simulink model "bdot_simple_sim"  (R2016b)
settings: Solver=VariableStepAuto  StartTime=0.0  StopTime=10000  RelTol=1e-3  EnableMultiTasking=on
values from neighbouring files (symbols this model uses):
  fsw_params = init_fsw_params()    [bdot_controller_edit_test.m]    (also in bdot_controlller_unit_test.m)
  sim_params = init_sim_params(fsw_params)    [bdot_controller_edit_test.m]    (also in bdot_controlller_unit_test.m)
undefined symbols (not defined in the file or in its folder): DiscIntNeverNeededParam
libraries: aerolibutil x5, vrlib x1, bdot_controller_lib x1, magnetorquer_assembly_lib x1
settings Model: Creator=Taylor  LastModifiedBy=taylorreynolds
settings OptimizationCC: LifeSpan=inf
settings DebuggingCC: SFUnexpectedBacktrackingDiag=warning  SFNoUnconditionalDefaultTransitionDiag=warning  SFExecutionAtInitializationDiag=none
settings GRTTargetCC: TargetLangStandard=C89/C90 (ANSI)  GeneratePreprocessorConditionals=Disable all
settings ConfigComp: CovMetricSettings=dw  CovHtmlReporting=on  CovSaveCumulativeToWorkspaceVar=on  CovSaveSingleToWorkspaceVar=on  CovExternalEMLEnable=off

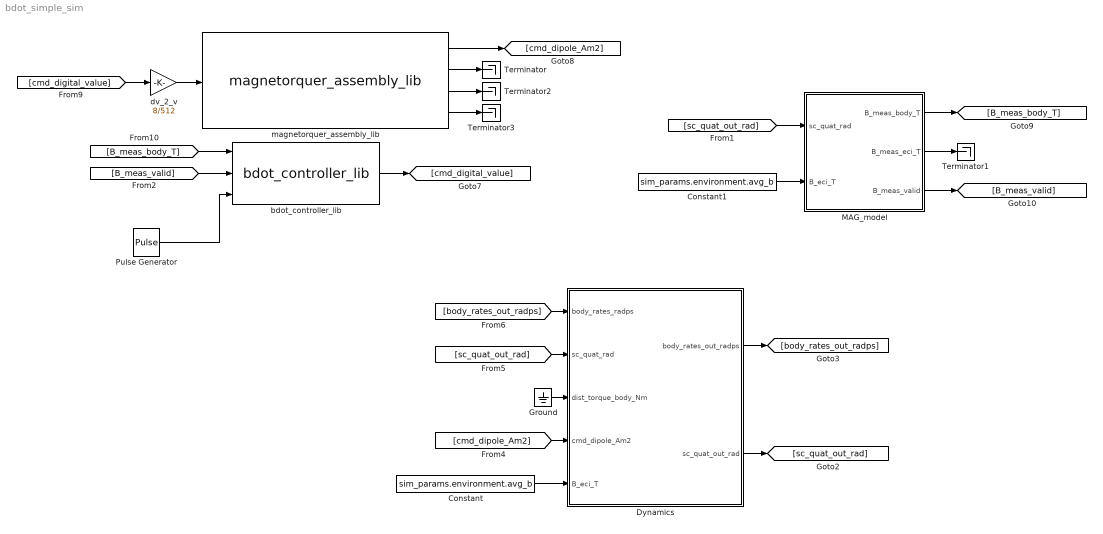
== system bdot_simple_sim ==
  Constant : Constant  Value=sim_params.environment.avg_b
  Constant1 : Constant  Value=sim_params.environment.avg_b
  Dynamics : Subsystem
  Ground : Ground
  MAG_model : Subsystem
  Pulse Generator : DiscretePulseGenerator  PulseType=Time based  Period=1  PulseWidth=sim_params.actuators.magnetorquer.actuation_time_pct
  Terminator{,1..3} (4 alike) : Terminator
  bdot_controller_lib : bdot_controller_lib/bdot_controller_lib
  dv_2_v : Gain  Gain=8/512
  magnetorquer_assembly_lib : magnetorquer_assembly_lib/magnetorquer_assembly_lib
  wires:
  bdot_controller_lib/1 -> [cmd_digital_value]
  [B_meas_body_T] -> bdot_controller_lib/1
  MAG_model/3(B_meas_valid) -> [B_meas_valid]
  MAG_model/1(B_meas_body_T) -> [B_meas_body_T]
  MAG_model/2(B_meas_eci_T) -> Terminator1/1
  [sc_quat_out_rad] -> MAG_model/1(sc_quat_rad)
  Constant1/1 -> MAG_model/2(B_eci_T)
  [body_rates_out_radps] -> Dynamics/1(body_rates_radps)
  Dynamics/1(body_rates_out_radps) -> [body_rates_out_radps]
  Dynamics/2(sc_quat_out_rad) -> [sc_quat_out_rad]
  [sc_quat_out_rad] -> Dynamics/2(sc_quat_rad)
  Ground/1 -> Dynamics/3(dist_torque_body_Nm)
  [cmd_dipole_Am2] -> Dynamics/4(cmd_dipole_Am2)
  Constant/1 -> Dynamics/5(B_eci_T)
  [B_meas_valid] -> bdot_controller_lib/2
  Pulse Generator/1 -> bdot_controller_lib/3
  dv_2_v/1 -> magnetorquer_assembly_lib/1
  [cmd_digital_value] -> dv_2_v/1
  magnetorquer_assembly_lib/1 -> [cmd_dipole_Am2]
  magnetorquer_assembly_lib/2 -> Terminator/1
  magnetorquer_assembly_lib/4 -> Terminator3/1
  magnetorquer_assembly_lib/3 -> Terminator2/1

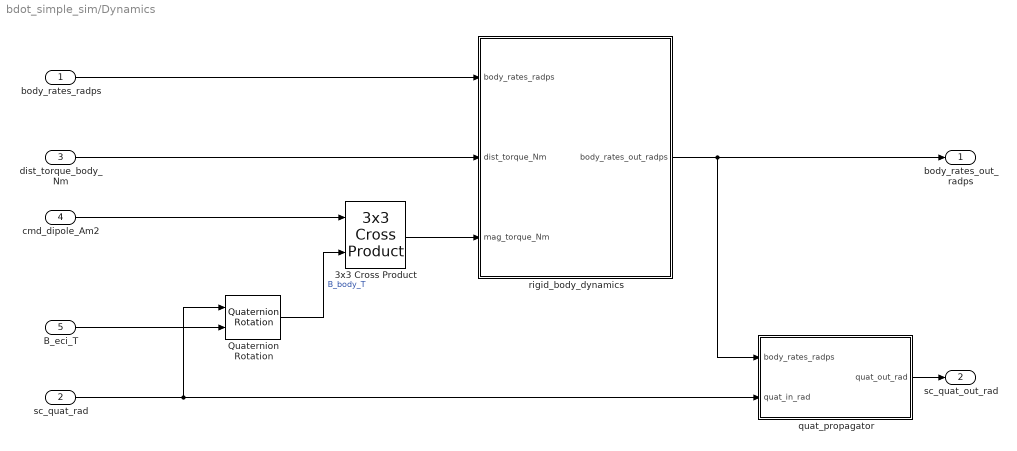
== system bdot_simple_sim/Dynamics ==
  body_rates_radps : Inport
  sc_quat_rad : Inport  Port=2
  dist_torque_body_Nm : Inport  Port=3
  cmd_dipole_Am2 : Inport  Port=4
  B_eci_T : Inport  Port=5
  3x3 Cross Product : aerolibutil/3x3 Cross Product
  Quaternion Rotation : aerolibutil/Quaternion Rotation
  quat_propagator : Subsystem
  rigid_body_dynamics : Subsystem
  body_rates_out_radps : Outport
  sc_quat_out_rad : Outport  Port=2
  wires:
  Quaternion Rotation/1 -> 3x3 Cross Product/2  "B_body_T"
  cmd_dipole_Am2/1 -> 3x3 Cross Product/1
  dist_torque_body_Nm/1 -> rigid_body_dynamics/2(dist_torque_Nm)
  sc_quat_rad/1 -> Quaternion Rotation/1, quat_propagator/2(quat_in_rad)
  quat_propagator/1(quat_out_rad) -> sc_quat_out_rad/1
  body_rates_radps/1 -> rigid_body_dynamics/1(body_rates_radps)
  rigid_body_dynamics/1(body_rates_out_radps) -> body_rates_out_radps/1, quat_propagator/1(body_rates_radps)
  B_eci_T/1 -> Quaternion Rotation/2
  3x3 Cross Product/1 -> rigid_body_dynamics/3(mag_torque_Nm)

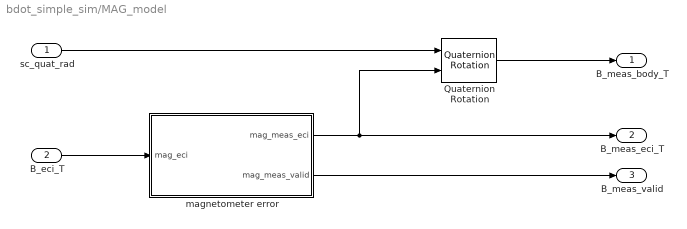
== system bdot_simple_sim/MAG_model ==
  sc_quat_rad : Inport
  B_eci_T : Inport  Port=2
  Quaternion Rotation : aerolibutil/Quaternion Rotation
  magnetometer error : Subsystem
  B_meas_body_T : Outport
  B_meas_eci_T : Outport  Port=2
  B_meas_valid : Outport  Port=3
  wires:
  sc_quat_rad/1 -> Quaternion Rotation/1
  B_eci_T/1 -> magnetometer error/1(mag_eci)
  magnetometer error/1(mag_meas_eci) -> Quaternion Rotation/2, B_meas_eci_T/1
  Quaternion Rotation/1 -> B_meas_body_T/1
  magnetometer error/2(mag_meas_valid) -> B_meas_valid/1

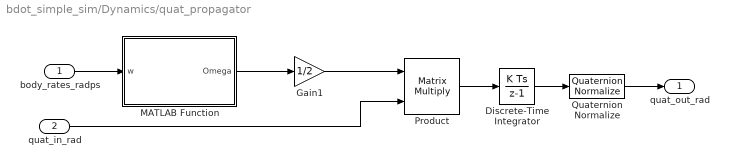
== system bdot_simple_sim/Dynamics/quat_propagator ==
  body_rates_radps : Inport
  quat_in_rad : Inport  Port=2
  Discrete-Time Integrator : DiscreteIntegrator  InitialCondition=sim_params.dynamics.ic.quat_init  InitialConditionSetting=State (most efficient)  SampleTime=fsw_params.sample_time_s  ICPrevOutput=DiscIntNeverNeededParam  ICPrevScaledInput=DiscIntNeverNeededParam
  Gain1 : Gain  Gain=1/2
  MATLAB Function : MATLAB Function  TreatAsAtomicUnit=on
  Product : Product  Multiplication=Matrix(*)  RndMeth=Zero
  Quaternion Normalize : aerolibutil/Quaternion Normalize
  quat_out_rad : Outport
  wires:
  Product/1 -> Discrete-Time Integrator/1
  Quaternion Normalize/1 -> quat_out_rad/1
  Discrete-Time Integrator/1 -> Quaternion Normalize/1
  Gain1/1 -> Product/1
  quat_in_rad/1 -> Product/2
  body_rates_radps/1 -> MATLAB Function/1(w)
  MATLAB Function/1(Omega) -> Gain1/1

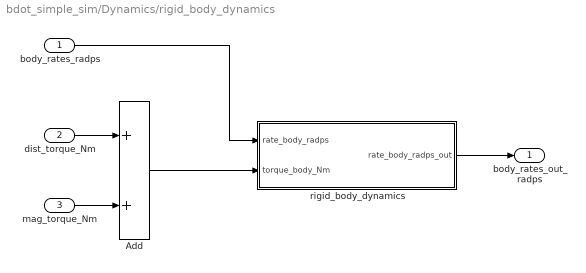
== system bdot_simple_sim/Dynamics/rigid_body_dynamics ==
  body_rates_radps : Inport
  dist_torque_Nm : Inport  Port=2
  mag_torque_Nm : Inport  Port=3
  Add : Sum
  rigid_body_dynamics : Subsystem
  body_rates_out_radps : Outport
  wires:
  dist_torque_Nm/1 -> Add/1
  Add/1 -> rigid_body_dynamics/2(torque_body_Nm)
  mag_torque_Nm/1 -> Add/2
  rigid_body_dynamics/1(rate_body_radps_out) -> body_rates_out_radps/1
  body_rates_radps/1 -> rigid_body_dynamics/1(rate_body_radps)

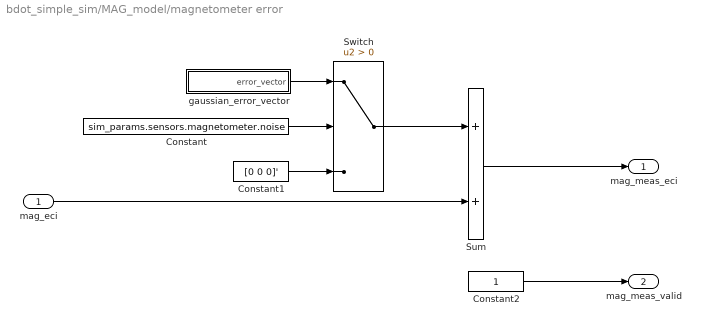
== system bdot_simple_sim/MAG_model/magnetometer error ==
  mag_eci : Inport
  Constant : Constant  Value=sim_params.sensors.magnetometer.noise
  Constant1 : Constant  Value=[0 0 0]'
  Constant2 : Constant
  Sum : Sum
  Switch : Switch  Criteria=u2 > Threshold
  gaussian_error_vector : Subsystem
  mag_meas_eci : Outport
  mag_meas_valid : Outport  Port=2
  wires:
  Constant2/1 -> mag_meas_valid/1
  Switch/1 -> Sum/1
  Constant1/1 -> Switch/3
  Constant/1 -> Switch/2
  gaussian_error_vector/1(error_vector) -> Switch/1
  Sum/1 -> mag_meas_eci/1
  mag_eci/1 -> Sum/2

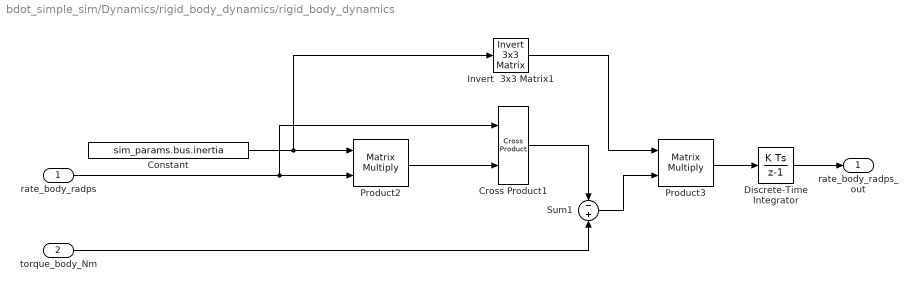
== system bdot_simple_sim/Dynamics/rigid_body_dynamics/rigid_body_dynamics ==
  rate_body_radps : Inport
  torque_body_Nm : Inport  Port=2
  Constant : Constant  Value=sim_params.bus.inertia
  Cross Product1 : vrlib/Utilities/Cross Product
  Discrete-Time Integrator : DiscreteIntegrator  InitialCondition=sim_params.dynamics.ic.rate_init  InitialConditionSetting=State (most efficient)  SampleTime=fsw_params.sample_time_s  ICPrevOutput=DiscIntNeverNeededParam  ICPrevScaledInput=DiscIntNeverNeededParam
  Invert  3x3 Matrix1 : aerolibutil/Invert  3x3 Matrix
  Product2 : Product  Multiplication=Matrix(*)  RndMeth=Zero
  Product3 : Product  Multiplication=Matrix(*)  RndMeth=Zero
  Sum1 : Sum  Inputs=-+
  rate_body_radps_out : Outport
  wires:
  Discrete-Time Integrator/1 -> rate_body_radps_out/1
  Product3/1 -> Discrete-Time Integrator/1
  Invert  3x3 Matrix1/1 -> Product3/1
  Sum1/1 -> Product3/2
  torque_body_Nm/1 -> Sum1/2
  Cross Product1/1 -> Sum1/1
  rate_body_radps/1 -> Product2/2, Cross Product1/1
  Product2/1 -> Cross Product1/2
  Constant/1 -> Product2/1, Invert  3x3 Matrix1/1

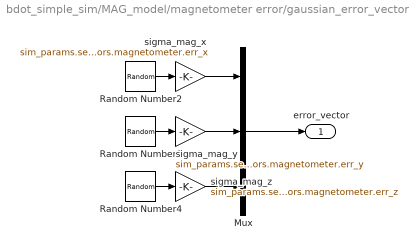
== system bdot_simple_sim/MAG_model/magnetometer error/gaussian_error_vector ==
  Mux : Mux  Inputs=3
  Random Number2 : RandomNumber  SampleTime=sim_params.sensors.magnetometer.sample_time_s
  Random Number3 : RandomNumber  Seed=1  SampleTime=sim_params.sensors.magnetometer.sample_time_s
  Random Number4 : RandomNumber  Seed=2  SampleTime=sim_params.sensors.magnetometer.sample_time_s
  sigma_mag_x : Gain  Gain=sim_params.sensors.magnetometer.err_x
  sigma_mag_y : Gain  Gain=sim_params.sensors.magnetometer.err_y
  sigma_mag_z : Gain  Gain=sim_params.sensors.magnetometer.err_z
  error_vector : Outport
  wires:
  Random Number2/1 -> sigma_mag_x/1
  Random Number4/1 -> sigma_mag_z/1
  Random Number3/1 -> sigma_mag_y/1
  sigma_mag_x/1 -> Mux/1
  sigma_mag_y/1 -> Mux/2
  Mux/1 -> error_vector/1
  sigma_mag_z/1 -> Mux/3

== matlab function bdot_simple_sim/Dynamics/quat_propagator/MATLAB Function ==
  data: w input; Omega output
function Omega = skew_sym(w)
%#codegen

    w_skew = ...
        [0 w(3) -w(2);
        -w(3) 0 w(1);
        w(2) -w(1) 0];

    Omega = ...
        [0 -w';
        w w_skew];
